simulink subsystem "Subsystem_LEDStrip"  (R2021b)
settings: Solver=VariableStepAuto  StartTime=0.0  StopTime=10.0  RelTol=1e-3
undefined symbols (not defined in the file): LED_OptPow, MLED_Vth
libraries: ee_lib x8, fl_lib x4, nesl_utility x3
settings Model: Creator=vlenzi  LastModifiedBy=vlenzi
settings SolverCC: AlgebraicLoopSolver=TrustRegion
settings DebuggingCC: SFMachineParentedDataDiag=warning

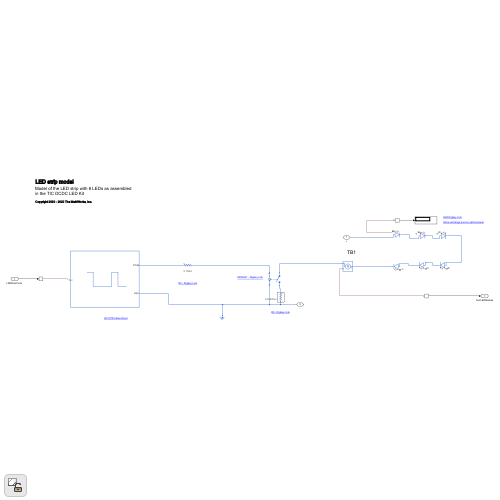
[thumbnail: Simulink's stored preview of the top-level diagram]
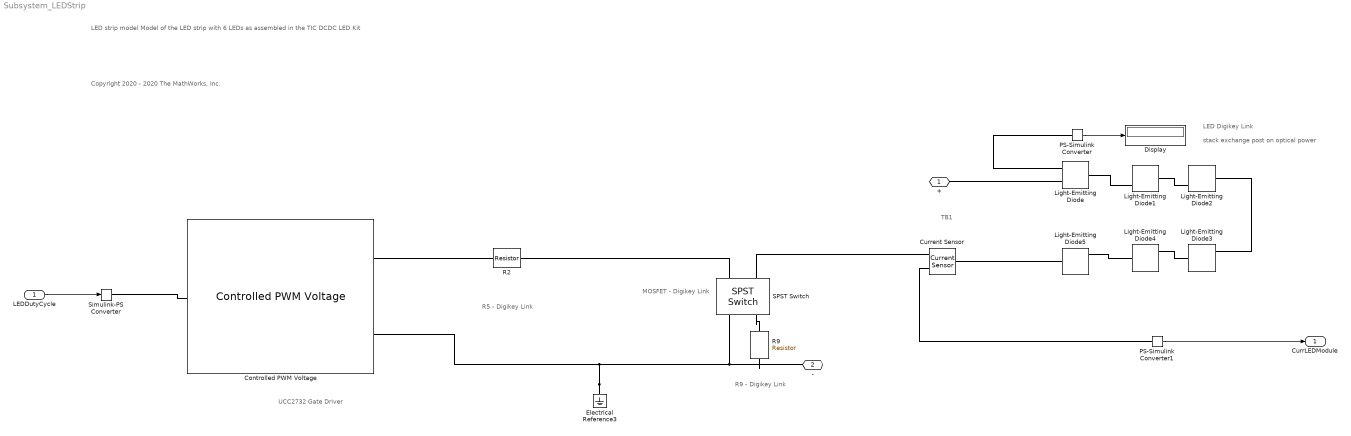
== system Subsystem_LEDStrip ==
  note: UCC2732 Gate Driver
  note: MOSFET - Digikey Link
  note: stack exchange post on optical power
  note: LED Digikey Link
  note: R9 - Digikey Link
  note: TB1
  note: R5 - Digikey Link
  note: LED strip model
      | Model of the LED strip with 6 LEDs as assembled in the TIC DCDC LED Kit
  note: Copyright 2020 - 2020 The MathWorks, Inc.
  LEDDutyCycle : Inport
  Controlled PWM Voltage : ee_lib/Integrated Circuits/Controlled PWM Voltage  F=FPWMLEDs Hz  TD=0 s  pulse_width_offset=0 s  pulse_min=0 s  pwm_or_av=1  event_type=1  sample_time=1e-6 s  Vmin=0 V  Vmax=5 V  Vm=12 V  u_min=0  u_max=1
      settings: InternalSimscapePortConfiguration="{\"Bottom\":[],\"Left\":[{\"id\":\"u\",\"label\":\"u\",\"type\":\"input\"}],\"Right\":[{\"id\":\"p2\",\"label\":\"PWM\",\"type\":\"foundation.electrical.electrical\"},{\"id\":\"n2\",\"label\":\"REF\",\"type\":\"foundation.electrical.electrical\"}],\"Top\":[]}"
  Current Sensor : fl_lib/Electrical/Electrical Sensors/Current Sensor
  Display : Display
  Electrical Reference3 : fl_lib/Electrical/Electrical Elements/Electrical Reference
  Light-Emitting Diode{,1..5} (6 alike) : ee_lib/Sensors & Transducers/Light-Emitting Diode  Gain=LED_OptPow W/A  prmExp=1  I12=LED_If A  V12=LED_Vf V  IS=5e-5 A  ec=10  RS=LED_Rs Ohm  Tmeas=LED_Temp degC  C_param=1  CJ=0 pF  CJ0=20 pF  VJ=1 V  Mgrad=0.5  Vvec=[.1, 10, 100] V  Cvec=[15, 10, 2] pF  FC=0.5  T_param=1  IS_T2=1.8e-4 A  I1_T2=0.0034 A  V1_T2=1.05 V  Tmeas2=125 degC  EG_param=1  EG=1.11 eV  XTI_param=1  XTI=3  Tdevice=25 degC  i_capacitor_specify=off  i_capacitor_priority=High  i_capacitor=0 A  i_capacitor_nominal_specify=off  i_capacitor_nominal_unit=A  i_capacitor_nominal_value=1  v_capacitor_specify=off  v_capacitor_priority=None  v_capacitor=0 V  v_capacitor_nominal_specify=off  v_capacitor_nominal_unit=V  v_capacitor_nominal_value=1  thermal_network_parameterization=ee.enum.thermalNetworkTopology.junctionCase  Rth=[0, 10] K/W  Rth_Cauer=[1, 3, 10] K/W  Rth_Foster=[4, 6] K/W  thermal_mass_parameterization=ee.enum.thermalNetwork.timeconstant  thermal_mass=[0, 1] J/K  thermal_mass_Cauer=[1.5, 2, 3] J/K  thermal_mass_Foster=[1.5, 3] J/K  thermal_time_constant=[0, 10] s  thermal_time_constant_Cauer=[1, 3, 10] s  thermal_time_constant_Foster=[6, 18] s  thermal_mass_initial_temperatures=[25, 25] degC  thermal_mass_initial_temperatures_Cauer=[25, 25, 25] degC  steadyState_Foster=simscape.enum.onoff.on  Tvec_initial_Foster=[25, 25, 25, 25] degC
      settings: SourceProductBaseCode=PS  InternalSimscapePortConfiguration="{\"Bottom\":[],\"Left\":[{\"id\":\"W\",\"label\":\"W\",\"type\":\"output\"},{\"id\":\"p\",\"label\":\"\",\"type\":\"foundation.electrical.electrical\"}],\"Right\":[{\"id\":\"n\",\"label\":\"\",\"type\":\"foundation.electrical.electrical\"}],\"Top\":[]}"
  PS-Simulink Converter : nesl_utility/PS-Simulink Converter  PhysicalDomain=network_engine_domain  SubClassName=ps_output  LeftPortType=input  RightPortType=output  PseudoPeriodic=off  Frequencies=[]  Unit=inherit  AffineConversion=off
      settings: SourceProductBaseCode=PW,SS
  PS-Simulink Converter1 : nesl_utility/PS-Simulink Converter  PhysicalDomain=network_engine_domain  SubClassName=ps_output  LeftPortType=input  RightPortType=output  PseudoPeriodic=off  Frequencies=[]  Unit=mA  AffineConversion=off
      settings: SourceProductBaseCode=PW,SS
  R2 : fl_lib/Electrical/Electrical Elements/Resistor  R=5.1 Ohm  i_specify=off  i_priority=None  i=0 A  i_nominal_specify=off  i_nominal_unit=A  i_nominal_value=1  v_specify=off  v_priority=None  v=0 V  v_nominal_specify=off  v_nominal_unit=V  v_nominal_value=1
      settings: AttributesFormatString=%<R>%<R_unit>
  R9 : fl_lib/Electrical/Electrical Elements/Resistor  R=0.250 Ohm  i_specify=off  i_priority=None  i=0 A  i_nominal_specify=off  i_nominal_unit=A  i_nominal_value=1  v_specify=off  v_priority=None  v=0 V  v_nominal_specify=off  v_nominal_unit=V  v_nominal_value=1
      settings: AttributesFormatString=%<R>%<R_unit>
  SPST Switch : ee_lib/Switches & Breakers/SPST Switch  R_closed=MLED_Rds Ohm  G_open=1e-6 S  Threshold=MLED_Vth V  Width=0 V  model_dynamics=0  t_on=1e-3 s  t_off=1e-3 s  initial_vT=0 V
      settings: SourceProductBaseCode=PS  InternalSimscapePortConfiguration="{\"Bottom\":[],\"Left\":[{\"id\":\"vTp\",\"label\":\"+\",\"type\":\"foundation.electrical.electrical\"},{\"id\":\"p\",\"label\":\"\",\"type\":\"foundation.electrical.electrical\"}],\"Right\":[{\"id\":\"vTn\",\"label\":\"-\",\"type\":\"foundation.electrical.electrical\"},{\"id\":\"n\",\"label\":\"\",\"type\":\"foundation.electrical.electrical\"}],\"Top\":[]}"
  Simulink-PS Converter : nesl_utility/Simulink-PS Converter  PhysicalDomain=network_engine_domain  SubClassName=ps_input  LeftPortType=input  RightPortType=output  PseudoPeriodic=off  Frequencies=[]  NoiseDistribution=none  NoiseParameters=[]  Unit=1  AffineConversion=off  FilteringAndDerivatives=provide  SimscapeFilterOrder=1  InputFilterTimeConstant=0.001  UdotUserProvided=0
      settings: SourceProductBaseCode=PW,SS
  + : PMIOPort  Side=Left
  - : PMIOPort  Port=2  Side=Right
  CurrLEDModule : Outport
  wires:
  PS-Simulink Converter/1 -> Display/1
  LEDDutyCycle/1 -> Simulink-PS Converter/1
  PS-Simulink Converter1/1 -> CurrLEDModule/1
  connections:
  Electrical Reference3/LConn1 -- -/RConn1 -- R9/RConn1 -- SPST Switch/RConn1 -- Controlled PWM Voltage/RConn2
  SPST Switch/LConn2 -- Current Sensor/RConn2
  SPST Switch/LConn1 -- R2/RConn1
  Light-Emitting Diode3/LConn2 -- Light-Emitting Diode2/RConn1
  Light-Emitting Diode2/LConn2 -- Light-Emitting Diode1/RConn1
  PS-Simulink Converter1/LConn1 -- Current Sensor/RConn1
  SPST Switch/RConn2 -- R9/LConn1
  Light-Emitting Diode4/LConn2 -- Light-Emitting Diode3/RConn1
  Light-Emitting Diode5/LConn2 -- Light-Emitting Diode4/RConn1
  Light-Emitting Diode/LConn1 -- PS-Simulink Converter/LConn1
  Controlled PWM Voltage/RConn1 -- R2/LConn1
  Light-Emitting Diode/LConn2 -- +/RConn1
  Light-Emitting Diode/RConn1 -- Light-Emitting Diode1/LConn2
  Light-Emitting Diode5/RConn1 -- Current Sensor/LConn1
  Simulink-PS Converter/RConn1 -- Controlled PWM Voltage/LConn1
